simulink model "2(B)"  (R2019b)
settings: Solver=VariableStepAuto  StartTime=0.0  StopTime=10.0  RelTol=1e-3
settings Model: Creator=tracy  LastModifiedBy=tracy

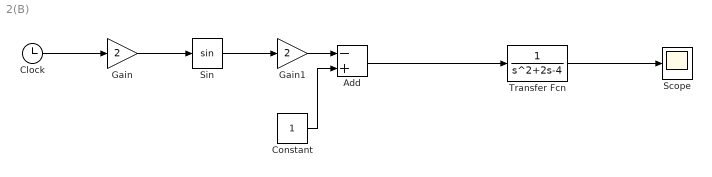
== system 2(B) ==
  Add : Sum  Inputs=-+
  Clock : Clock
  Constant : Constant
  Gain : Gain  Gain=2
  Gain1 : Gain  Gain=2
  Scope : Scope
  Sin : Trigonometry
  Transfer Fcn : TransferFcn  Denominator=[1 2 -4]
  wires:
  Clock/1 -> Gain/1
  Constant/1 -> Add/2
  Gain1/1 -> Add/1
  Sin/1 -> Gain1/1
  Gain/1 -> Sin/1
  Add/1 -> Transfer Fcn/1
  Transfer Fcn/1 -> Scope/1
